simulink model "reducefun_verification"  (R2018a)
settings: Solver=VariableStepAuto  StartTime=0.0  StopTime=5  FixedStep=0.0001  RelTol=1e-3
values from neighbouring files (symbols this model uses):
  A_lat = [0 0.0535820961816 0 0 0 -0.28461980439 -32.1133643261 9.99720570373 1 0.0354985232569 -3.25227271927 -0.0202694214621 ... (16 elements, 4x4)]    [redu_ss.mat]    (also in redu_ss_openloop.mat; reducefun_openloop.m = A_lat_ac)
  A_lateral_lo = [0 0 0 0.0535820961816 0 0 0 0 0 0 0 0 ... (81 elements, 9x9)]    [sep_lofi_ss_openloop.mat]
  A_lon = [0 -32.1699999995 -3.8860153007e-13 0 0 -0.0122159649604 -0.000177990738877 -8.90562755929e-19 0 10.1727450892 -0.900587999136 -2.63777761256 ... (16 elements, 4x4)]    [redu_ss.mat]    (also in redu_ss_openloop.mat; reducefun_openloop.m = A_lon_ac)
  A_longitude_lo = [0 0 0.00011472600432 1.67159666407e-06 8.36370331111e-21 0 0 599.99999999 0 -32.1699999995 -3.8860153007e-13 0 ... (49 elements, 7x7)]    [sep_lofi_ss_openloop.mat]
  B_lat = [0  0; 0.000242601411088  0.000712015887462; -0.761094183546  0.115332321948; -0.0449043309427  -0.0788692177557]    [redu_ss.mat]    (also in redu_ss_openloop.mat; reducefun_openloop.m = B_lat_ac)
  B_lateral_lo = [0 0 0 0 0 0 1 0 0 0 0 0 ... (27 elements, 9x3)]    [sep_lofi_ss_openloop.mat]
  B_lon = [0 0.184926492709 -0.00189996119559 -0.192753630035]    [redu_ss.mat]    (also in redu_ss_openloop.mat; reducefun_openloop.m = B_lon_ac)
  B_longitude_lo = [0 0 0 0 0 1 0 0 0 0 0 0 ... (14 elements, 7x2)]    [sep_lofi_ss_openloop.mat]
  C_lat = [57.2957795131 0 0 0 0 57.2957795131 0 0 0 0 57.2957795131 0 ... (16 elements, 4x4)]    [redu_ss.mat]    (also in redu_ss_openloop.mat; reducefun_openloop.m = C_lat_ac)
  C_lateral_lo = [57.2957795131 0 0 0 0 0 0 57.2957795131 0 0 0 0 ... (54 elements, 6x9)]    [sep_lofi_ss_openloop.mat]
  C_lon = [57.2957795131 0 0 0 0 1 0 0 0 0 57.2957795131 0 ... (16 elements, 4x4)]    [redu_ss.mat]    (also in redu_ss_openloop.mat; reducefun_openloop.m = C_lon_ac)
  C_longitude_lo = [1 0 0 0 0 0 57.2957795131 0 0 0 0 0 ... (35 elements, 5x7)]    [sep_lofi_ss_openloop.mat]
  D_lat = [0  0; 0  0; 0  0; 0  0]    [redu_ss.mat]    (also in redu_ss_openloop.mat; reducefun_openloop.m = D_lat_ac)
  D_lateral_lo = [0 0 0 0 0 0 0 0 0 0 0 0 ... (18 elements, 6x3)]    [sep_lofi_ss_openloop.mat]
  D_lon = [0 0 0 0]    [redu_ss.mat]    (also in redu_ss_openloop.mat; reducefun_openloop.m = D_lon_ac)
  D_longitude_lo = [0  0; 0  0; 0  0; 0  0; 0  0]    [sep_lofi_ss_openloop.mat]
settings Model: Creator=Lukas  LastModifiedBy=Lukas

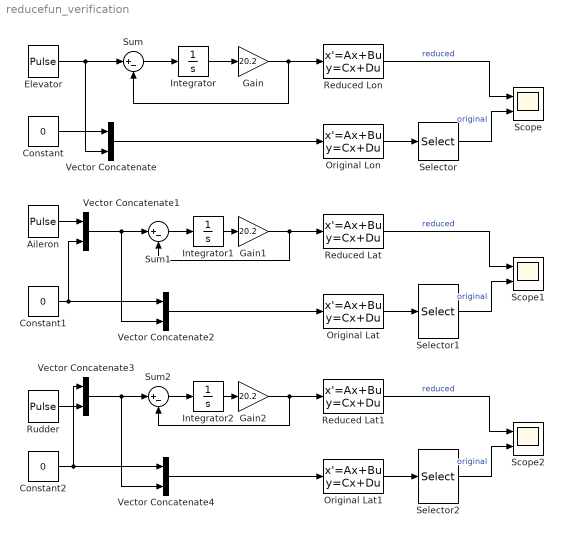
== system reducefun_verification ==
  Aileron : DiscretePulseGenerator  PulseType=Time based  Amplitude=0.025  Period=10  PulseWidth=5
  Constant : Constant  Value=0
  Constant1 : Constant  Value=0
  Constant2 : Constant  Value=0
  Elevator : DiscretePulseGenerator  PulseType=Time based  Amplitude=0.025  Period=10  PulseWidth=5
  Gain : Gain  Gain=20.2
  Gain1 : Gain  Gain=20.2
  Gain2 : Gain  Gain=20.2
  Integrator : Integrator
  Integrator1 : Integrator
  Integrator2 : Integrator
  Original Lat : StateSpace  A=A_lateral_lo  B=B_lateral_lo  C=C_lateral_lo  D=D_lateral_lo  InitialCondition=0
  Original Lat1 : StateSpace  A=A_lateral_lo  B=B_lateral_lo  C=C_lateral_lo  D=D_lateral_lo  InitialCondition=0
  Original Lon : StateSpace  A=A_longitude_lo  B=B_longitude_lo  C=C_longitude_lo  D=D_longitude_lo  InitialCondition=0
  Reduced Lat : StateSpace  A=A_lat  B=B_lat  C=C_lat  D=D_lat  InitialCondition=0
  Reduced Lat1 : StateSpace  A=A_lat  B=B_lat  C=C_lat  D=D_lat  InitialCondition=0
  Reduced Lon : StateSpace  A=A_lon  B=B_lon  C=C_lon  D=D_lon  InitialCondition=0
  Rudder : DiscretePulseGenerator  PulseType=Time based  Amplitude=0.025  Period=10  PulseWidth=5
  Scope : Scope  NumInputPorts=2
  Scope1 : Scope  NumInputPorts=2
  Scope2 : Scope  NumInputPorts=2
  Selector : Selector  InputPortWidth=5  IndexOptions=Index vector (dialog)  Indices=[2 3 4 5]  OutputSizes=1
  Selector1 : Selector  InputPortWidth=6  IndexOptions=Index vector (dialog)  Indices=[1 4 5 6]  OutputSizes=1
  Selector2 : Selector  InputPortWidth=6  IndexOptions=Index vector (dialog)  Indices=[1 4 5 6]  OutputSizes=1
  Sum : Sum  Inputs=|+-
  Sum1 : Sum  Inputs=|+-
  Sum2 : Sum  Inputs=|+-
  Vector Concatenate{,1..4} (5 alike) : Concatenate
  wires:
  Gain/1 -> Reduced Lon/1, Sum/2
  Sum/1 -> Integrator/1
  Reduced Lon/1 -> Scope/1  "reduced"
  Elevator/1 -> Vector Concatenate/2, Sum/1
  Gain1/1 -> Sum1/2, Reduced Lat/1
  Vector Concatenate/1 -> Original Lon/1
  Constant/1 -> Vector Concatenate/1
  Vector Concatenate2/1 -> Original Lat/1
  Vector Concatenate1/1 -> Vector Concatenate2/2, Sum1/1
  Aileron/1 -> Vector Concatenate1/1
  Constant1/1 -> Vector Concatenate2/1, Vector Concatenate1/2
  Integrator/1 -> Gain/1
  Sum1/1 -> Integrator1/1
  Integrator1/1 -> Gain1/1
  Original Lon/1 -> Selector/1
  Selector/1 -> Scope/2  "original"
  Sum2/1 -> Integrator2/1
  Constant2/1 -> Vector Concatenate3/1, Vector Concatenate4/1
  Vector Concatenate3/1 -> Vector Concatenate4/2, Sum2/1
  Gain2/1 -> Sum2/2, Reduced Lat1/1
  Vector Concatenate4/1 -> Original Lat1/1
  Integrator2/1 -> Gain2/1
  Rudder/1 -> Vector Concatenate3/2
  Selector1/1 -> Scope1/2  "original"
  Original Lat/1 -> Selector1/1
  Reduced Lat/1 -> Scope1/1  "reduced"
  Reduced Lat1/1 -> Scope2/1  "reduced"
  Original Lat1/1 -> Selector2/1
  Selector2/1 -> Scope2/2  "original"
